simulink model "triphase_filter"  (R2015a)
settings: Solver=ode45  StartTime=0.0  StopTime=10.0  RelTol=1e-3
values from neighbouring files (symbols this model uses):
  Ts = 1/fs    (= 2e-06)    [VOC_param.m]    (also in VOC_param_paper.m = 5e-05; controller_parameters.m = 5e-05; power_control_param.m = 1e-05)
undefined symbols (not defined in the file or in its folder): fdesignblkfcn, gcbh
settings Model: Creator=rblan  LastModifiedBy=rblan

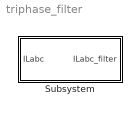
== system triphase_filter ==
  Subsystem : Subsystem

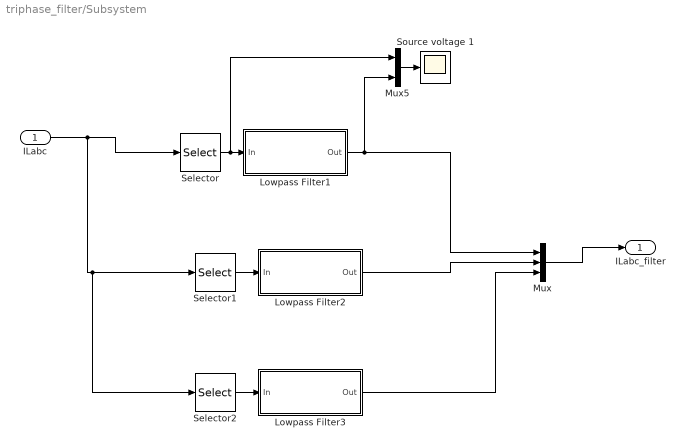
== system triphase_filter/Subsystem ==
  ILabc : Inport
  Lowpass Filter1 : Subsystem  DialogController=fdesignblkfcn  InitFcn=fdesignblkfcn(gcbh, {'InitFcn'});  mask(Lowpass Filter){}
      mask help: Design a lowpass filter
      settings: CopyFcn=fdesignblkfcn(gcbh, {'CopyFcn'});
      mask Help: helpview(mapfilelocation('dsp'), 'dsplowpassfilter');
      mask Display: disp('Lowpass')
  Lowpass Filter2 : Subsystem  DialogController=fdesignblkfcn  InitFcn=fdesignblkfcn(gcbh, {'InitFcn'});  mask(Lowpass Filter){}
      mask help: Design a lowpass filter
      settings: CopyFcn=fdesignblkfcn(gcbh, {'CopyFcn'});
      mask Help: helpview(mapfilelocation('dsp'), 'dsplowpassfilter');
      mask Display: disp('Lowpass')
  Lowpass Filter3 : Subsystem  DialogController=fdesignblkfcn  InitFcn=fdesignblkfcn(gcbh, {'InitFcn'});  mask(Lowpass Filter){}
      mask help: Design a lowpass filter
      settings: CopyFcn=fdesignblkfcn(gcbh, {'CopyFcn'});
      mask Help: helpview(mapfilelocation('dsp'), 'dsplowpassfilter');
      mask Display: disp('Lowpass')
  Mux : Mux  Inputs=3
  Mux5 : Mux  Inputs=2
  Selector : Selector  InputPortWidth=3  Indices=[1 ]
  Selector1 : Selector  InputPortWidth=3  Indices=[2 ]
  Selector2 : Selector  InputPortWidth=3  Indices=[3 ]
  Source voltage 1 : Scope
      settings: TimeRange=0.06239913932221623  YMin=-20  YMax=20  SaveName=Uabc3
  "ILabc_filter " : Outport
  wires:
  Selector/1 -> Mux5/1, Lowpass Filter1/1(In)
  Selector1/1 -> Lowpass Filter2/1(In)
  Selector2/1 -> Lowpass Filter3/1(In)
  ILabc/1 -> Selector2/1, Selector1/1, Selector/1
  Mux/1 -> "ILabc_filter "/1
  Lowpass Filter1/1(Out) -> Mux5/2, Mux/1
  Lowpass Filter2/1(Out) -> Mux/2
  Lowpass Filter3/1(Out) -> Mux/3
  Mux5/1 -> Source voltage 1/1

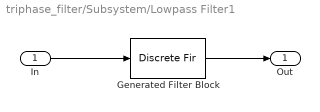
== system triphase_filter/Subsystem/Lowpass Filter1 ==
  In : Inport
  Generated Filter Block : DiscreteFir  Tag=BlockMethodSubSystem  Coefficients=[0.00066997061007102146 0.00039594753768134921 0.00050923833364043838 0.00064121023987765411 0.00079280782867979847 0.00096565195948745096 0.0011612249134648441 0.0013813034112891537 0.0016258363797603168 0.00189586775152624 0.0021937967665738986 0.0025182856156895374 0.0028712153581181305 0.0032524075930221406 0.0036619213302328162 0.0040995922875411367 0.0045647115037281407 0.0050571693774376092 0.0055755644713608998 0.0061188755386402038 0.0066858046869813807 0.0072743876095049858 0.0078826151797070851 0.008508279928147176 0.0091487654418524397 0.0098015587445344776 0.010463408044883112 0.011131631365616724 0.01180255916983277 0.012472923323742597 0.013138965213669168 0.013797128508656864 0.014443472674505006 0.015074413551179873 0.015686005300183669 0.016274804762768966 0.016836841850885544 0.017368928902123198 0.017867353313765707 0.018329137210770056 0.01875098545282421 0.019130337105350597 0.019464385406778938 0.019751100568202895 0.01998827113369786 0.020174555288683272 0.020308392586653162 0.020389170733429815 0.020416063050480212 0.020389170733429815 0.020308392586653162 0.020174555288683272 0.01998827113369786 0.019751100568202895 0.019464385406778938 0.019130337105350597 0.01875098545282421 0.018329137210770056 0.017867353313765707 0.017368928902123198 0.016836841850885544 0.016274804762768966 0.015686005300183669 0.015074413551179873 0.014443472674505006 0.013797128508656864 0.013138965213669168 0.012472923323742597 0.01180255916983277 0.011131631365616724 0.010463408044883112 0.0098015587445344776 0.0091487654418524397 0.008508279928147176 0.0078826151797070851 0.0072743876095049858 0.0066858046869813807 0.0061188755386402038 0.0055755644713608998 0.0050571693774376092 0.0045647115037281407 0.0040995922875411367 0.0036619213302328162 0.0032524075930221406 0.0028712153581181305 0.0025182856156895374 0.0021937967665738986 0.00189586775152624 0.0016258363797603168 0.0013813034112891537 0.0011612249134648441 0.00096565195948745096 0.00079280782867979847 0.00064121023987765411 0.00050923833364043838 0.00039594753768134921 0.00066997061007102146]  InputProcessing=Columns as channels (frame based)  SampleTime=Ts
  Out : Outport
  wires:
  In/1 -> Generated Filter Block/1
  Generated Filter Block/1 -> Out/1

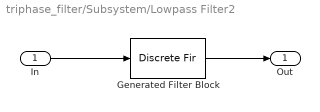
== system triphase_filter/Subsystem/Lowpass Filter2 ==
  In : Inport
  Generated Filter Block : DiscreteFir  Tag=BlockMethodSubSystem  Coefficients=[0.00066997061007102146 0.00039594753768134921 0.00050923833364043838 0.00064121023987765411 0.00079280782867979847 0.00096565195948745096 0.0011612249134648441 0.0013813034112891537 0.0016258363797603168 0.00189586775152624 0.0021937967665738986 0.0025182856156895374 0.0028712153581181305 0.0032524075930221406 0.0036619213302328162 0.0040995922875411367 0.0045647115037281407 0.0050571693774376092 0.0055755644713608998 0.0061188755386402038 0.0066858046869813807 0.0072743876095049858 0.0078826151797070851 0.008508279928147176 0.0091487654418524397 0.0098015587445344776 0.010463408044883112 0.011131631365616724 0.01180255916983277 0.012472923323742597 0.013138965213669168 0.013797128508656864 0.014443472674505006 0.015074413551179873 0.015686005300183669 0.016274804762768966 0.016836841850885544 0.017368928902123198 0.017867353313765707 0.018329137210770056 0.01875098545282421 0.019130337105350597 0.019464385406778938 0.019751100568202895 0.01998827113369786 0.020174555288683272 0.020308392586653162 0.020389170733429815 0.020416063050480212 0.020389170733429815 0.020308392586653162 0.020174555288683272 0.01998827113369786 0.019751100568202895 0.019464385406778938 0.019130337105350597 0.01875098545282421 0.018329137210770056 0.017867353313765707 0.017368928902123198 0.016836841850885544 0.016274804762768966 0.015686005300183669 0.015074413551179873 0.014443472674505006 0.013797128508656864 0.013138965213669168 0.012472923323742597 0.01180255916983277 0.011131631365616724 0.010463408044883112 0.0098015587445344776 0.0091487654418524397 0.008508279928147176 0.0078826151797070851 0.0072743876095049858 0.0066858046869813807 0.0061188755386402038 0.0055755644713608998 0.0050571693774376092 0.0045647115037281407 0.0040995922875411367 0.0036619213302328162 0.0032524075930221406 0.0028712153581181305 0.0025182856156895374 0.0021937967665738986 0.00189586775152624 0.0016258363797603168 0.0013813034112891537 0.0011612249134648441 0.00096565195948745096 0.00079280782867979847 0.00064121023987765411 0.00050923833364043838 0.00039594753768134921 0.00066997061007102146]  InputProcessing=Columns as channels (frame based)  SampleTime=Ts
  Out : Outport
  wires:
  In/1 -> Generated Filter Block/1
  Generated Filter Block/1 -> Out/1

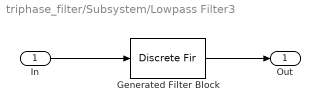
== system triphase_filter/Subsystem/Lowpass Filter3 ==
  In : Inport
  Generated Filter Block : DiscreteFir  Tag=BlockMethodSubSystem  Coefficients=[0.00066997061007102146 0.00039594753768134921 0.00050923833364043838 0.00064121023987765411 0.00079280782867979847 0.00096565195948745096 0.0011612249134648441 0.0013813034112891537 0.0016258363797603168 0.00189586775152624 0.0021937967665738986 0.0025182856156895374 0.0028712153581181305 0.0032524075930221406 0.0036619213302328162 0.0040995922875411367 0.0045647115037281407 0.0050571693774376092 0.0055755644713608998 0.0061188755386402038 0.0066858046869813807 0.0072743876095049858 0.0078826151797070851 0.008508279928147176 0.0091487654418524397 0.0098015587445344776 0.010463408044883112 0.011131631365616724 0.01180255916983277 0.012472923323742597 0.013138965213669168 0.013797128508656864 0.014443472674505006 0.015074413551179873 0.015686005300183669 0.016274804762768966 0.016836841850885544 0.017368928902123198 0.017867353313765707 0.018329137210770056 0.01875098545282421 0.019130337105350597 0.019464385406778938 0.019751100568202895 0.01998827113369786 0.020174555288683272 0.020308392586653162 0.020389170733429815 0.020416063050480212 0.020389170733429815 0.020308392586653162 0.020174555288683272 0.01998827113369786 0.019751100568202895 0.019464385406778938 0.019130337105350597 0.01875098545282421 0.018329137210770056 0.017867353313765707 0.017368928902123198 0.016836841850885544 0.016274804762768966 0.015686005300183669 0.015074413551179873 0.014443472674505006 0.013797128508656864 0.013138965213669168 0.012472923323742597 0.01180255916983277 0.011131631365616724 0.010463408044883112 0.0098015587445344776 0.0091487654418524397 0.008508279928147176 0.0078826151797070851 0.0072743876095049858 0.0066858046869813807 0.0061188755386402038 0.0055755644713608998 0.0050571693774376092 0.0045647115037281407 0.0040995922875411367 0.0036619213302328162 0.0032524075930221406 0.0028712153581181305 0.0025182856156895374 0.0021937967665738986 0.00189586775152624 0.0016258363797603168 0.0013813034112891537 0.0011612249134648441 0.00096565195948745096 0.00079280782867979847 0.00064121023987765411 0.00050923833364043838 0.00039594753768134921 0.00066997061007102146]  InputProcessing=Columns as channels (frame based)  SampleTime=Ts
  Out : Outport
  wires:
  In/1 -> Generated Filter Block/1
  Generated Filter Block/1 -> Out/1
